simulink model "test"  (R2013a)
settings: Solver=ode45  StartTime=0.0  StopTime=5.0  RelTol=1e-3
undefined symbols (not defined in the file or in its folder): viewMap
libraries: fuzblock x1
settings Model: Creator=Marek  LastModifiedBy=Marek

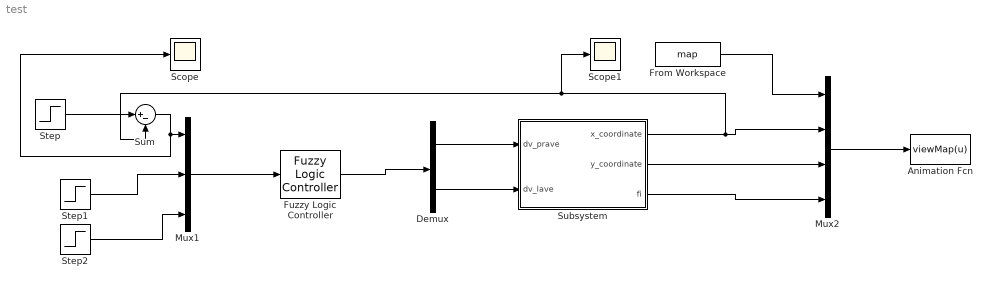
== system test ==
  Animation Fcn : MATLABFcn  MATLABFcn=viewMap(u)  OutputDimensions=0  SampleTime=0.01
  Demux : Demux  Outputs=2
  From Workspace : FromWorkspace  VariableName=map  SampleTime=0
  Fuzzy Logic Controller : fuzblock/Fuzzy Logic  Controller  fis=fuzcar
  Mux1 : Mux  Inputs=3
  Mux2 : Mux
  Scope : Scope
  Scope1 : Scope
  Step : Step  Time=0  Before=5  After=0  SampleTime=0
  Step1 : Step  Time=0  After=0.5  SampleTime=0
  Step2 : Step  Time=0  After=0.5  SampleTime=0
  Subsystem : Subsystem
  Sum : Sum  Inputs=|+-
  wires:
  Step/1 -> Sum/1
  Step1/1 -> Mux1/2
  Mux1/1 -> Fuzzy Logic Controller/1
  Fuzzy Logic Controller/1 -> Demux/1
  Demux/1 -> Subsystem/1(dv_prave)
  Demux/2 -> Subsystem/2(dv_lave)
  Subsystem/1(x_coordinate) -> Scope1/1, Sum/2, Mux2/2
  Subsystem/2(y_coordinate) -> Mux2/3
  Subsystem/3("fi ") -> Mux2/4
  Mux2/1 -> Animation Fcn/1
  Step2/1 -> Mux1/3
  From Workspace/1 -> Mux2/1
  Sum/1 -> Scope/1, Mux1/1

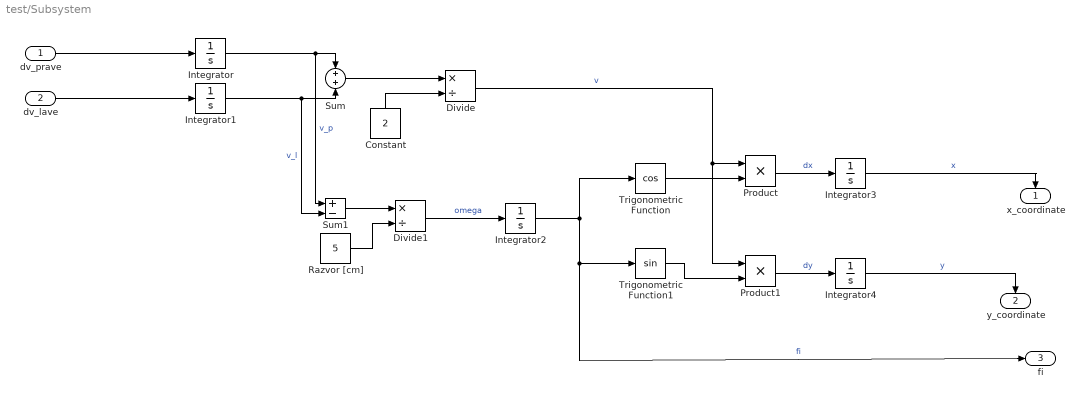
== system test/Subsystem ==
  dv_prave : Inport
  dv_lave : Inport  Port=2
  Constant : Constant  Value=2
  Divide : Product  Inputs=*/
  Divide1 : Product  Inputs=*/
  Integrator : Integrator
  Integrator1 : Integrator
  Integrator2 : Integrator  InitialCondition=45
  Integrator3 : Integrator  InitialCondition=10
  Integrator4 : Integrator  InitialCondition=10
  Product : Product
  Product1 : Product
  Razvor [cm] : Constant  Value=5
  Sum : Sum
  Sum1 : Sum  Inputs=+-
  Trigonometric Function : Trigonometry  Operator=cos
  Trigonometric Function1 : Trigonometry
  x_coordinate : Outport
  y_coordinate : Outport  Port=2
  "fi " : Outport  Port=3
  wires:
  Divide/1 -> Product/1, Product1/1  "v"
  Integrator1/1 -> Sum1/2, Sum/2  "v_l"
  Integrator/1 -> Sum1/1, Sum/1  "v_p"
  Constant/1 -> Divide/2
  Trigonometric Function/1 -> Product/2
  Integrator2/1 -> "fi "/1, Trigonometric Function1/1, Trigonometric Function/1  "fi"
  Product1/1 -> Integrator4/1  "dy"
  Sum/1 -> Divide/1
  Product/1 -> Integrator3/1  "dx"
  Trigonometric Function1/1 -> Product1/2
  dv_prave/1 -> Integrator/1
  Integrator3/1 -> x_coordinate/1  "x"
  dv_lave/1 -> Integrator1/1
  Sum1/1 -> Divide1/1
  Divide1/1 -> Integrator2/1  "omega"
  Razvor [cm]/1 -> Divide1/2
  Integrator4/1 -> y_coordinate/1  "y"
